simulink model "Exp1_pendulum_model2022a"  (R2022a)
settings: Solver=VariableStepAuto  StartTime=0.0  StopTime=10.0  RelTol=1e-3
values from neighbouring files (symbols this model uses):
  d = m * g * l * (cos(phi_2) - cos(phi_1)) / Integral    [Exp1_estimation_d.m]    (also in Exp1_parameters_steel_math.m = 0.00266991944412; Exp1_parameters_steel_phys.m = 0.00274110004552; Exp1_parameters_styrofoam_math.m = 0.000186312591304; Exp1_parameters_styrofoam_phys.m = 0.00166165647764)
  J = m*l^2    (= 0.4942189)    [Exp1_parameters_steel_math.m]    (also in Exp1_parameters_steel_phys.m = 0.503352452; Exp1_parameters_styrofoam_math.m = 0.0016639175; Exp1_parameters_styrofoam_phys.m = 0.0101157325)
undefined symbols (not defined in the file or in its folder): Fgl, omega_0, phi_0
settings Model: Creator=shaunclarenceraj  LastModifiedBy=shaunclarenceraj
settings ModelReferenceCC: EnableRefExpFcnMdlSchedulingChecks=off
settings RTWCC: Description=Generic Real-Time Target

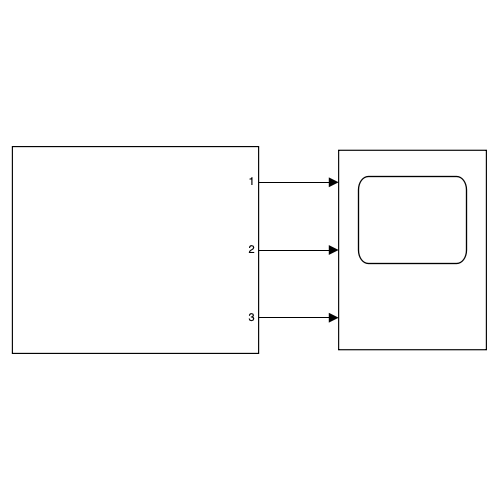
[thumbnail: Simulink's stored preview of the top-level diagram]
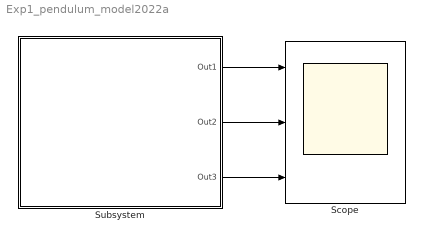
== system Exp1_pendulum_model2022a ==
  Scope : Scope  NumInputPorts=3
  Subsystem : Subsystem
  wires:
  Subsystem/1(Out1) -> Scope/1
  Subsystem/2(Out2) -> Scope/2
  Subsystem/3(Out3) -> Scope/3

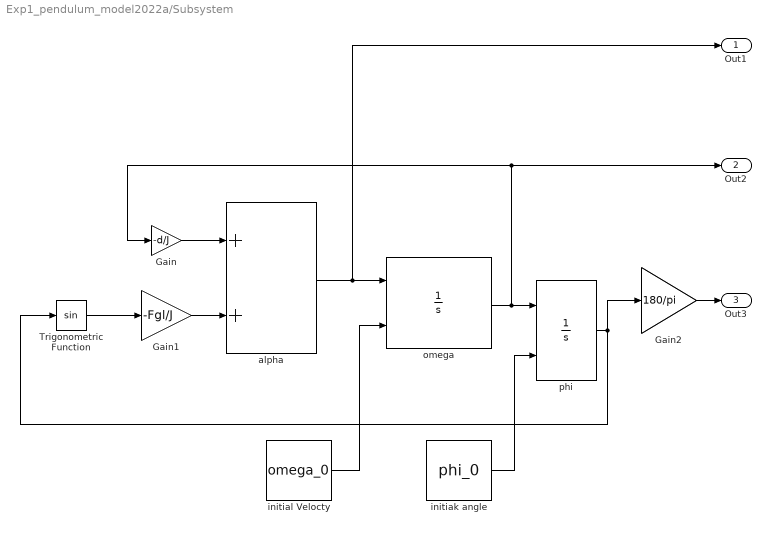
== system Exp1_pendulum_model2022a/Subsystem ==
  Gain : Gain  Gain=-d/J
  Gain1 : Gain  Gain=-Fgl/J
  Gain2 : Gain  Gain=180/pi
  Trigonometric Function : Trigonometry
  alpha : Sum
  initiak angle : Constant  Value=phi_0
  "initial Velocty " : Constant  Value=omega_0
  omega : Integrator  InitialConditionSource=external
  phi : Integrator  InitialConditionSource=external
  Out1 : Outport
  Out2 : Outport  Port=2
  Out3 : Outport  Port=3
  wires:
  alpha/1 -> omega/1, Out1/1
  "initial Velocty "/1 -> omega/2
  Gain/1 -> alpha/1
  Gain1/1 -> alpha/2
  phi/1 -> Gain2/1, Trigonometric Function/1
  omega/1 -> Out2/1, Gain/1, phi/1
  Gain2/1 -> Out3/1
  Trigonometric Function/1 -> Gain1/1
  initiak angle/1 -> phi/2
